simulink model "SWC_VES_type"  (R2021b)
settings: Solver=FixedStepDiscrete  StartTime=0.0  StopTime=10.0  FixedStep=0.001  RelTol=1e-3
undefined symbols (not defined in the file or in its folder): R_HALINCDD_CSOP_IPCF_Handler
libraries: simulink x78
(part 2 of 2)

== system SWC_VES_type/run_Trig_IpcfDataReceive_sys/Write_TBOX1/RLDWdwCtrlCmd ==
  Byte_9 : Inport
  BitwiseAND : simulink/Logic and Bit Operations/Bitwise Operator  logicop=AND  UseBitMask=off  NumInputPorts=2  BitMask=bin2dec('11011001')  BitMaskRealWorld=Stored Integer
  BitwiseOR : simulink/Logic and Bit Operations/Bitwise Operator  logicop=OR  UseBitMask=off  BitMask=bin2dec('11011001')  BitMaskRealWorld=Stored Integer
  Constant : Constant  Value=(2^7-1)
  LeftShift : ArithShift  BitShiftDirection=Left
  RightShift : ArithShift  BitShiftDirection=Right
  UnitConverter : DataTypeConversion  OutDataTypeStr=uint8
  UnitConverter1 : DataTypeConversion  OutDataTypeStr=uint8
  VHAL_RLDWdwCtrlCmd_cnt : Outport
  wires:
  Byte_9/1 -> UnitConverter1/1
  UnitConverter1/1 -> LeftShift/1
  LeftShift/1 -> BitwiseOR/1
  BitwiseAND/1 -> VHAL_RLDWdwCtrlCmd_cnt/1
  Constant/1 -> UnitConverter/1
  UnitConverter/1 -> BitwiseAND/2
  RightShift/1 -> BitwiseAND/1
  BitwiseOR/1 -> RightShift/1

== system SWC_VES_type/run_Trig_IpcfDataReceive_sys/Write_TBOX1/RRDWdwCtrlCmd ==
  Byte_10 : Inport
  BitwiseAND : simulink/Logic and Bit Operations/Bitwise Operator  logicop=AND  UseBitMask=off  NumInputPorts=2  BitMask=bin2dec('11011001')  BitMaskRealWorld=Stored Integer
  BitwiseOR : simulink/Logic and Bit Operations/Bitwise Operator  logicop=OR  UseBitMask=off  BitMask=bin2dec('11011001')  BitMaskRealWorld=Stored Integer
  Constant : Constant  Value=(2^7-1)
  LeftShift : ArithShift  BitShiftDirection=Left
  RightShift : ArithShift  BitShiftDirection=Right
  UnitConverter : DataTypeConversion  OutDataTypeStr=uint8
  UnitConverter1 : DataTypeConversion  OutDataTypeStr=uint8
  VHAL_RRDWdwCtrlCmd_cnt : Outport
  wires:
  BitwiseOR/1 -> RightShift/1
  RightShift/1 -> BitwiseAND/1
  UnitConverter/1 -> BitwiseAND/2
  Constant/1 -> UnitConverter/1
  BitwiseAND/1 -> VHAL_RRDWdwCtrlCmd_cnt/1
  LeftShift/1 -> BitwiseOR/1
  UnitConverter1/1 -> LeftShift/1
  Byte_10/1 -> UnitConverter1/1

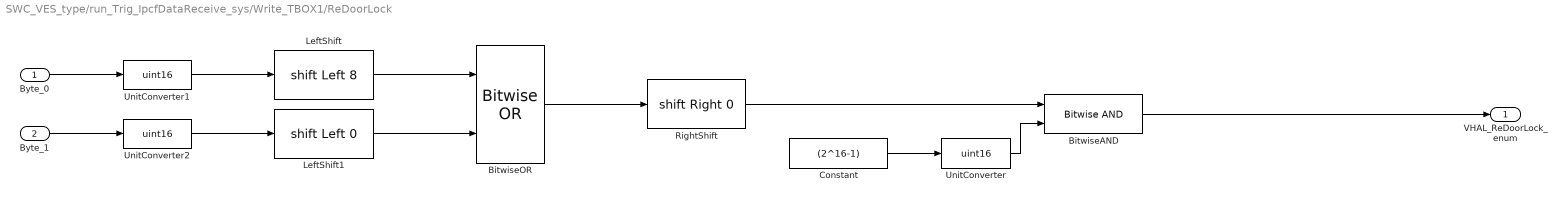
== system SWC_VES_type/run_Trig_IpcfDataReceive_sys/Write_TBOX1/ReDoorLock ==
  Byte_0 : Inport
  Byte_1 : Inport  Port=2
  BitwiseAND : simulink/Logic and Bit Operations/Bitwise Operator  logicop=AND  UseBitMask=off  NumInputPorts=2  BitMask=bin2dec('11011001')  BitMaskRealWorld=Stored Integer
  BitwiseOR : simulink/Logic and Bit Operations/Bitwise Operator  logicop=OR  UseBitMask=off  NumInputPorts=2  BitMask=bin2dec('11011001')  BitMaskRealWorld=Stored Integer
  Constant : Constant  Value=(2^16-1)
  LeftShift : ArithShift  BitShiftNumber=8  BitShiftDirection=Left
  LeftShift1 : ArithShift  BitShiftDirection=Left
  RightShift : ArithShift  BitShiftDirection=Right
  UnitConverter : DataTypeConversion  OutDataTypeStr=uint16
  UnitConverter1 : DataTypeConversion  OutDataTypeStr=uint16
  UnitConverter2 : DataTypeConversion  OutDataTypeStr=uint16
  VHAL_ReDoorLock_enum : Outport
  wires:
  BitwiseOR/1 -> RightShift/1
  RightShift/1 -> BitwiseAND/1
  UnitConverter/1 -> BitwiseAND/2
  Constant/1 -> UnitConverter/1
  BitwiseAND/1 -> VHAL_ReDoorLock_enum/1
  LeftShift/1 -> BitwiseOR/1
  UnitConverter1/1 -> LeftShift/1
  Byte_0/1 -> UnitConverter1/1
  LeftShift1/1 -> BitwiseOR/2
  UnitConverter2/1 -> LeftShift1/1
  Byte_1/1 -> UnitConverter2/1

== system SWC_VES_type/run_Trig_IpcfDataReceive_sys/Write_TBOX1/ReOutsideMirror ==
  Byte_5 : Inport
  BitwiseAND : simulink/Logic and Bit Operations/Bitwise Operator  logicop=AND  UseBitMask=off  NumInputPorts=2  BitMask=bin2dec('11011001')  BitMaskRealWorld=Stored Integer
  BitwiseOR : simulink/Logic and Bit Operations/Bitwise Operator  logicop=OR  UseBitMask=off  BitMask=bin2dec('11011001')  BitMaskRealWorld=Stored Integer
  Constant : Constant  Value=(2^2-1)
  LeftShift : ArithShift  BitShiftDirection=Left
  RightShift : ArithShift  BitShiftNumber=2  BitShiftDirection=Right
  UnitConverter : DataTypeConversion  OutDataTypeStr=uint8
  UnitConverter1 : DataTypeConversion  OutDataTypeStr=uint8
  VHAL_ReOutsideMirror_enum : Outport
  wires:
  BitwiseOR/1 -> RightShift/1
  RightShift/1 -> BitwiseAND/1
  UnitConverter/1 -> BitwiseAND/2
  Constant/1 -> UnitConverter/1
  BitwiseAND/1 -> VHAL_ReOutsideMirror_enum/1
  LeftShift/1 -> BitwiseOR/1
  UnitConverter1/1 -> LeftShift/1
  Byte_5/1 -> UnitConverter1/1

== system SWC_VES_type/run_Trig_IpcfDataReceive_sys/Write_TBOX1/RePwrReqTbox ==
  Byte_3 : Inport
  BitwiseAND : simulink/Logic and Bit Operations/Bitwise Operator  logicop=AND  UseBitMask=off  NumInputPorts=2  BitMask=bin2dec('11011001')  BitMaskRealWorld=Stored Integer
  BitwiseOR : simulink/Logic and Bit Operations/Bitwise Operator  logicop=OR  UseBitMask=off  BitMask=bin2dec('11011001')  BitMaskRealWorld=Stored Integer
  Constant : Constant  Value=(2^3-1)
  LeftShift : ArithShift  BitShiftDirection=Left
  RightShift : ArithShift  BitShiftNumber=5  BitShiftDirection=Right
  UnitConverter : DataTypeConversion  OutDataTypeStr=uint8
  UnitConverter1 : DataTypeConversion  OutDataTypeStr=uint8
  VHAL_RePwrReqTbox_enum : Outport
  wires:
  BitwiseOR/1 -> RightShift/1
  RightShift/1 -> BitwiseAND/1
  UnitConverter/1 -> BitwiseAND/2
  Constant/1 -> UnitConverter/1
  BitwiseAND/1 -> VHAL_RePwrReqTbox_enum/1
  LeftShift/1 -> BitwiseOR/1
  UnitConverter1/1 -> LeftShift/1
  Byte_3/1 -> UnitConverter1/1

== system SWC_VES_type/run_Trig_IpcfDataReceive_sys/Write_TBOX1/ReRadio ==
  Byte_6 : Inport
  BitwiseAND : simulink/Logic and Bit Operations/Bitwise Operator  logicop=AND  UseBitMask=off  NumInputPorts=2  BitMask=bin2dec('11011001')  BitMaskRealWorld=Stored Integer
  BitwiseOR : simulink/Logic and Bit Operations/Bitwise Operator  logicop=OR  UseBitMask=off  BitMask=bin2dec('11011001')  BitMaskRealWorld=Stored Integer
  Constant : Constant  Value=(2^1-1)
  LeftShift : ArithShift  BitShiftDirection=Left
  RightShift : ArithShift  BitShiftNumber=7  BitShiftDirection=Right
  UnitConverter : DataTypeConversion  OutDataTypeStr=uint8
  UnitConverter1 : DataTypeConversion  OutDataTypeStr=uint8
  VHAL_ReRadio_flg : Outport
  wires:
  BitwiseOR/1 -> RightShift/1
  RightShift/1 -> BitwiseAND/1
  UnitConverter/1 -> BitwiseAND/2
  Constant/1 -> UnitConverter/1
  BitwiseAND/1 -> VHAL_ReRadio_flg/1
  LeftShift/1 -> BitwiseOR/1
  UnitConverter1/1 -> LeftShift/1
  Byte_6/1 -> UnitConverter1/1

== system SWC_VES_type/run_Trig_IpcfDataReceive_sys/Write_TBOX1/RemoteACTemp ==
  Byte_7 : Inport
  BitwiseAND : simulink/Logic and Bit Operations/Bitwise Operator  logicop=AND  UseBitMask=off  NumInputPorts=2  BitMask=bin2dec('11011001')  BitMaskRealWorld=Stored Integer
  BitwiseOR : simulink/Logic and Bit Operations/Bitwise Operator  logicop=OR  UseBitMask=off  BitMask=bin2dec('11011001')  BitMaskRealWorld=Stored Integer
  Constant : Constant  Value=(2^6-1)
  LeftShift : ArithShift  BitShiftDirection=Left
  RightShift : ArithShift  BitShiftDirection=Right
  UnitConverter : DataTypeConversion  OutDataTypeStr=uint8
  UnitConverter1 : DataTypeConversion  OutDataTypeStr=uint8
  VHAL_RemoteACTemp_C : Outport
  wires:
  BitwiseOR/1 -> RightShift/1
  RightShift/1 -> BitwiseAND/1
  UnitConverter/1 -> BitwiseAND/2
  Constant/1 -> UnitConverter/1
  BitwiseAND/1 -> VHAL_RemoteACTemp_C/1
  LeftShift/1 -> BitwiseOR/1
  UnitConverter1/1 -> LeftShift/1
  Byte_7/1 -> UnitConverter1/1

== system SWC_VES_type/run_Trig_IpcfDataReceive_sys/Write_TBOX1/RemoteAutoReq ==
  Byte_7 : Inport
  BitwiseAND : simulink/Logic and Bit Operations/Bitwise Operator  logicop=AND  UseBitMask=off  NumInputPorts=2  BitMask=bin2dec('11011001')  BitMaskRealWorld=Stored Integer
  BitwiseOR : simulink/Logic and Bit Operations/Bitwise Operator  logicop=OR  UseBitMask=off  BitMask=bin2dec('11011001')  BitMaskRealWorld=Stored Integer
  Constant : Constant  Value=(2^1-1)
  LeftShift : ArithShift  BitShiftDirection=Left
  RightShift : ArithShift  BitShiftNumber=7  BitShiftDirection=Right
  UnitConverter : DataTypeConversion  OutDataTypeStr=uint8
  UnitConverter1 : DataTypeConversion  OutDataTypeStr=uint8
  VHAL_RemoteAutoReq_flg : Outport
  wires:
  BitwiseOR/1 -> RightShift/1
  RightShift/1 -> BitwiseAND/1
  UnitConverter/1 -> BitwiseAND/2
  Constant/1 -> UnitConverter/1
  BitwiseAND/1 -> VHAL_RemoteAutoReq_flg/1
  LeftShift/1 -> BitwiseOR/1
  UnitConverter1/1 -> LeftShift/1
  Byte_7/1 -> UnitConverter1/1

== system SWC_VES_type/run_Trig_IpcfDataReceive_sys/Write_TBOX1/RemoteMidAutoReq ==
  Byte_7 : Inport
  BitwiseAND : simulink/Logic and Bit Operations/Bitwise Operator  logicop=AND  UseBitMask=off  NumInputPorts=2  BitMask=bin2dec('11011001')  BitMaskRealWorld=Stored Integer
  BitwiseOR : simulink/Logic and Bit Operations/Bitwise Operator  logicop=OR  UseBitMask=off  BitMask=bin2dec('11011001')  BitMaskRealWorld=Stored Integer
  Constant : Constant  Value=(2^1-1)
  LeftShift : ArithShift  BitShiftDirection=Left
  RightShift : ArithShift  BitShiftNumber=6  BitShiftDirection=Right
  UnitConverter : DataTypeConversion  OutDataTypeStr=uint8
  UnitConverter1 : DataTypeConversion  OutDataTypeStr=uint8
  VHAL_RemoteMidAutoReq_flg : Outport
  wires:
  BitwiseOR/1 -> RightShift/1
  RightShift/1 -> BitwiseAND/1
  UnitConverter/1 -> BitwiseAND/2
  Constant/1 -> UnitConverter/1
  BitwiseAND/1 -> VHAL_RemoteMidAutoReq_flg/1
  LeftShift/1 -> BitwiseOR/1
  UnitConverter1/1 -> LeftShift/1
  Byte_7/1 -> UnitConverter1/1

== system SWC_VES_type/run_Trig_IpcfDataReceive_sys/Write_TBOX1/TBOXNETSIGSTR ==
  Byte_6 : Inport
  BitwiseAND : simulink/Logic and Bit Operations/Bitwise Operator  logicop=AND  UseBitMask=off  NumInputPorts=2  BitMask=bin2dec('11011001')  BitMaskRealWorld=Stored Integer
  BitwiseOR : simulink/Logic and Bit Operations/Bitwise Operator  logicop=OR  UseBitMask=off  BitMask=bin2dec('11011001')  BitMaskRealWorld=Stored Integer
  Constant : Constant  Value=(2^4-1)
  LeftShift : ArithShift  BitShiftDirection=Left
  RightShift : ArithShift  BitShiftNumber=4  BitShiftDirection=Right
  UnitConverter : DataTypeConversion  OutDataTypeStr=uint8
  UnitConverter1 : DataTypeConversion  OutDataTypeStr=uint8
  VHAL_TBOXNETSIGSTR_enum : Outport
  wires:
  BitwiseOR/1 -> RightShift/1
  RightShift/1 -> BitwiseAND/1
  UnitConverter/1 -> BitwiseAND/2
  Constant/1 -> UnitConverter/1
  BitwiseAND/1 -> VHAL_TBOXNETSIGSTR_enum/1
  LeftShift/1 -> BitwiseOR/1
  UnitConverter1/1 -> LeftShift/1
  Byte_6/1 -> UnitConverter1/1

== system SWC_VES_type/run_Trig_IpcfDataReceive_sys/Write_TBOX1/TBOXReDTCData ==
  Byte_5 : Inport
  BitwiseAND : simulink/Logic and Bit Operations/Bitwise Operator  logicop=AND  UseBitMask=off  NumInputPorts=2  BitMask=bin2dec('11011001')  BitMaskRealWorld=Stored Integer
  BitwiseOR : simulink/Logic and Bit Operations/Bitwise Operator  logicop=OR  UseBitMask=off  BitMask=bin2dec('11011001')  BitMaskRealWorld=Stored Integer
  Constant : Constant  Value=(2^2-1)
  LeftShift : ArithShift  BitShiftDirection=Left
  RightShift : ArithShift  BitShiftDirection=Right
  UnitConverter : DataTypeConversion  OutDataTypeStr=uint8
  UnitConverter1 : DataTypeConversion  OutDataTypeStr=uint8
  VHAL_TBOXReDTCData_enum : Outport
  wires:
  BitwiseOR/1 -> RightShift/1
  RightShift/1 -> BitwiseAND/1
  UnitConverter/1 -> BitwiseAND/2
  Constant/1 -> UnitConverter/1
  BitwiseAND/1 -> VHAL_TBOXReDTCData_enum/1
  LeftShift/1 -> BitwiseOR/1
  UnitConverter1/1 -> LeftShift/1
  Byte_5/1 -> UnitConverter1/1

== system SWC_VES_type/run_Trig_IpcfDataReceive_sys/Write_TBOX1/TBOXReVehData ==
  Byte_2 : Inport
  BitwiseAND : simulink/Logic and Bit Operations/Bitwise Operator  logicop=AND  UseBitMask=off  NumInputPorts=2  BitMask=bin2dec('11011001')  BitMaskRealWorld=Stored Integer
  BitwiseOR : simulink/Logic and Bit Operations/Bitwise Operator  logicop=OR  UseBitMask=off  BitMask=bin2dec('11011001')  BitMaskRealWorld=Stored Integer
  Constant : Constant  Value=(2^2-1)
  LeftShift : ArithShift  BitShiftDirection=Left
  RightShift : ArithShift  BitShiftNumber=2  BitShiftDirection=Right
  UnitConverter : DataTypeConversion  OutDataTypeStr=uint8
  UnitConverter1 : DataTypeConversion  OutDataTypeStr=uint8
  VHAL_TBOXReVehData_enum : Outport
  wires:
  BitwiseOR/1 -> RightShift/1
  RightShift/1 -> BitwiseAND/1
  UnitConverter/1 -> BitwiseAND/2
  Constant/1 -> UnitConverter/1
  BitwiseAND/1 -> VHAL_TBOXReVehData_enum/1
  LeftShift/1 -> BitwiseOR/1
  UnitConverter1/1 -> LeftShift/1
  Byte_2/1 -> UnitConverter1/1

== system SWC_VES_type/run_Trig_IpcfDataReceive_sys/Write_TBOX1/TBOXRemoteOn ==
  Byte_2 : Inport
  BitwiseAND : simulink/Logic and Bit Operations/Bitwise Operator  logicop=AND  UseBitMask=off  NumInputPorts=2  BitMask=bin2dec('11011001')  BitMaskRealWorld=Stored Integer
  BitwiseOR : simulink/Logic and Bit Operations/Bitwise Operator  logicop=OR  UseBitMask=off  BitMask=bin2dec('11011001')  BitMaskRealWorld=Stored Integer
  Constant : Constant  Value=(2^2-1)
  LeftShift : ArithShift  BitShiftDirection=Left
  RightShift : ArithShift  BitShiftDirection=Right
  UnitConverter : DataTypeConversion  OutDataTypeStr=uint8
  UnitConverter1 : DataTypeConversion  OutDataTypeStr=uint8
  VHAL_TBOXRemoteOn_enum : Outport
  wires:
  BitwiseOR/1 -> RightShift/1
  RightShift/1 -> BitwiseAND/1
  UnitConverter/1 -> BitwiseAND/2
  Constant/1 -> UnitConverter/1
  BitwiseAND/1 -> VHAL_TBOXRemoteOn_enum/1
  LeftShift/1 -> BitwiseOR/1
  UnitConverter1/1 -> LeftShift/1
  Byte_2/1 -> UnitConverter1/1

== system SWC_VES_type/run_Trig_IpcfDataReceive_sys/Write_TBOX1/TBOXRemotePW ==
  Byte_3 : Inport
  BitwiseAND : simulink/Logic and Bit Operations/Bitwise Operator  logicop=AND  UseBitMask=off  NumInputPorts=2  BitMask=bin2dec('11011001')  BitMaskRealWorld=Stored Integer
  BitwiseOR : simulink/Logic and Bit Operations/Bitwise Operator  logicop=OR  UseBitMask=off  BitMask=bin2dec('11011001')  BitMaskRealWorld=Stored Integer
  Constant : Constant  Value=(2^5-1)
  LeftShift : ArithShift  BitShiftDirection=Left
  RightShift : ArithShift  BitShiftDirection=Right
  UnitConverter : DataTypeConversion  OutDataTypeStr=uint8
  UnitConverter1 : DataTypeConversion  OutDataTypeStr=uint8
  VHAL_TBOXRemotePW_enum : Outport
  wires:
  BitwiseOR/1 -> RightShift/1
  RightShift/1 -> BitwiseAND/1
  UnitConverter/1 -> BitwiseAND/2
  Constant/1 -> UnitConverter/1
  BitwiseAND/1 -> VHAL_TBOXRemotePW_enum/1
  LeftShift/1 -> BitwiseOR/1
  UnitConverter1/1 -> LeftShift/1
  Byte_3/1 -> UnitConverter1/1

== system SWC_VES_type/run_Trig_IpcfDataReceive_sys/Write_TBOX1/TBOXTESTSTATUS ==
  Byte_6 : Inport
  BitwiseAND : simulink/Logic and Bit Operations/Bitwise Operator  logicop=AND  UseBitMask=off  NumInputPorts=2  BitMask=bin2dec('11011001')  BitMaskRealWorld=Stored Integer
  BitwiseOR : simulink/Logic and Bit Operations/Bitwise Operator  logicop=OR  UseBitMask=off  BitMask=bin2dec('11011001')  BitMaskRealWorld=Stored Integer
  Constant : Constant  Value=(2^4-1)
  LeftShift : ArithShift  BitShiftDirection=Left
  RightShift : ArithShift  BitShiftDirection=Right
  UnitConverter : DataTypeConversion  OutDataTypeStr=uint8
  UnitConverter1 : DataTypeConversion  OutDataTypeStr=uint8
  VHAL_TBOXTESTSTATUS_enum : Outport
  wires:
  BitwiseOR/1 -> RightShift/1
  RightShift/1 -> BitwiseAND/1
  UnitConverter/1 -> BitwiseAND/2
  Constant/1 -> UnitConverter/1
  BitwiseAND/1 -> VHAL_TBOXTESTSTATUS_enum/1
  LeftShift/1 -> BitwiseOR/1
  UnitConverter1/1 -> LeftShift/1
  Byte_6/1 -> UnitConverter1/1
